simulink model "rot_simu"  (R2024a)
settings: Solver=VariableStepAuto  StartTime=0.0  StopTime=10.0  RelTol=1e-3
InitFcn:
  | m=10;
  | k=100;
  | r=0.05;
settings Model: LastModifiedBy=ximen

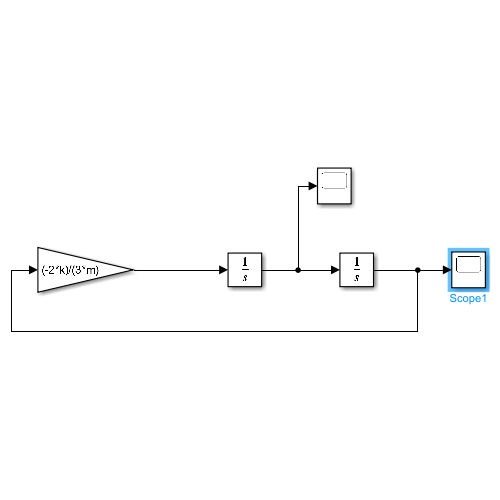
[thumbnail: Simulink's stored preview of the top-level diagram]
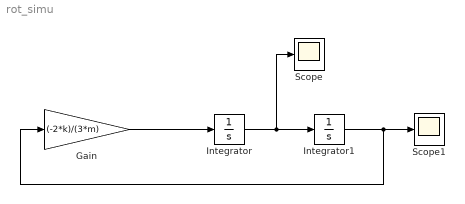
== system rot_simu ==
  Gain : Gain  Gain=(-2*k)/(3*m)
  Integrator : Integrator  InitialCondition=2
  Integrator1 : Integrator
  Scope : Scope
  Scope1 : Scope
  wires:
  Integrator/1 -> Scope/1, Integrator1/1
  Gain/1 -> Integrator/1
  Integrator1/1 -> Gain/1, Scope1/1
